simulink model "corner_detection_2019b_modified"  (R2022b)
settings: Solver=FixedStepDiscrete  StartTime=0.0  StopTime=0  RelTol=1e-3  EnableMultiTasking=on
undefined symbols (not defined in the file or in its folder): fspecial, gray, Rec, SDTV
libraries: visionsources x2, visionconversions x1, visionanalysis x1, visiontextngfix x1
settings Model: PacingRate=0.001800  Creator=FxMain  LastModifiedBy=User
settings SolverCC: AlgebraicLoopSolver=TrustRegion
settings DataIOCC: LimitDataPoints=on  SaveFormat=Array  ReturnWorkspaceOutputs=off
settings OptimizationCC: ExpressionDepthLimit=2147483647  LifeSpan=inf
settings DebuggingCC: UnderspecifiedInitializationDetection=Classic  MergeDetectMultiDrivingBlocksExec=none  SolverPrmCheckMsg=warning  FcnCallInpInsideContextMsg=warning  UnconnectedInputMsg=warning  UnconnectedOutputMsg=warning  UnconnectedLineMsg=warning  StateNameClashWarn=warning  SFUnexpectedBacktrackingDiag=warning  SFNoUnconditionalDefaultTransitionDiag=warning  SFExecutionAtInitializationDiag=none  SFMachineParentedDataDiag=warning  ArithmeticOperatorsInVariantConditions=warning
settings HardwareCC: ProdBitPerPointer=32  ProdBitPerSizeT=32  ProdBitPerPtrDiffT=32  ProdLargestAtomicFloat=None  ProdIntDivRoundTo=Undefined  ProdEndianess=Unspecified  ProdWordSize=32  ProdHWDeviceType=32-bit Generic
settings ModelReferenceCC: EnableRefExpFcnMdlSchedulingChecks=on  PropagateSignalLabelsOutOfModel=off
settings SFSimCC: SimUseLocalCustomCode=off  CustomCodeUndefinedFunction=UseInterfaceOnly
settings RTWCC: RTWUseLocalCustomCode=off
settings CodeAppCC: StateflowObjectComments=on
settings GRTTargetCC: TargetLangStandard=C89/C90 (ANSI)  CombineOutputUpdateFcns=off  GRTInterface=on
settings ConfigComp: CovMetricSettings=dw  CovSaveCumulativeToWorkspaceVar=on  CovSaveSingleToWorkspaceVar=on  CovExternalEMLEnable=off

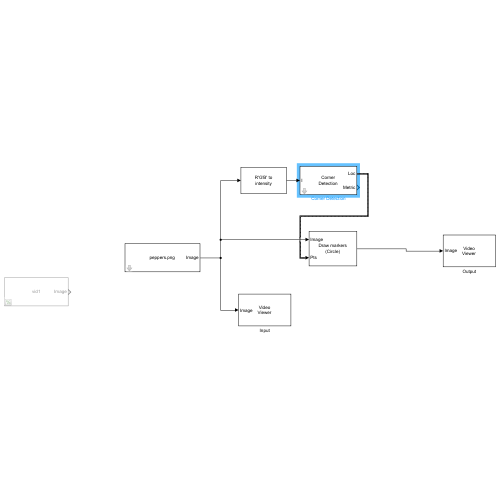
[thumbnail: Simulink's stored preview of the top-level diagram]
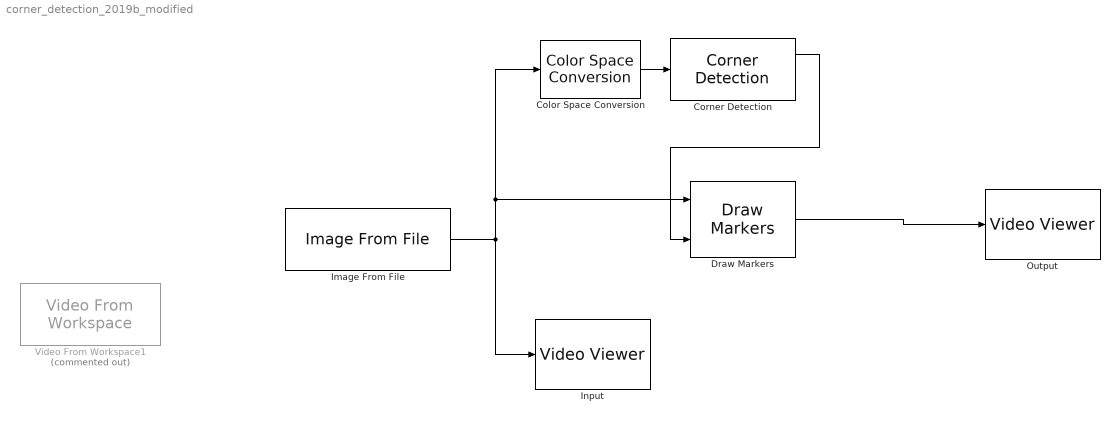
== system corner_detection_2019b_modified ==
  Color Space Conversion : visionconversions/Color Space  Conversion  conversion=Obsolete  conversionActive=R'G'B' to intensity  wp_str=D65  rec=Rec. 601 (SDTV)  sys=1125/60/2:1  imagePorts=One multidimensional signal
  Corner Detection : visionanalysis/Corner Detection  method=Local intensity comparison (Rosen & Drummond)  factor=0.02  filter=fspecial('gaussian', [1 5], 1.5)  thrInten=0.1  thrAngle=157.5  output=Obsolete9b  outputInUse=Corner location and metric matrix  maxNum=300  thrMetric=0.0005  neighborSize=[11 11]  isOutVarDim=on  roundingMode=Floor  overflowMode=off  firstCoeffMode=Specify word length  firstCoeffWordLength=16  firstCoeffFracLength=16  prodOutputMode=Binary point scaling  prodOutputWordLength=32  prodOutputFracLength=0  accumMode=Binary point scaling  accumWordLength=32  accumFracLength=0  memoryMode=Binary point scaling  memoryWordLength=32  memoryFracLength=0
  Draw Markers : visiontextngfix/Draw Markers  shape=Circle  size=20  fill=on  fillClrSource=Specify via dialog  display=White  intensity=200  color=255  opacity=0.6  viewport=Entire image  antialiasing=off  inType=Obsolete  imagePorts=One multidimensional signal  roundingMode=Floor  overflowMode=off  memoryMode=Specify word length  memoryWordLength=16  memoryFracLength=15  prodOutputMode=Binary point scaling  prodOutputWordLength=32  prodOutputFracLength=14
  Image From File : visionsources/Image From File  Tag=vipblks_nd  FileName=peppers.png  Ts=inf  imagePorts=One multidimensional signal  OutPortLabels=R|G|B  ImageDataType=Inherit from input image  sdImageDataType=uint(8)  Signed=on  WordLength=16  FractionLengthMode=User-defined  FractionLength=15
  Input : VideoViewer  colormapValue=gray(256)  FigPos=[141.8 567.6 519.2 385.6]
  Output : VideoViewer  colormapValue=gray(256)  FigPos=[663.4 573.2 520 384.8]
  Video From Workspace1 : visionsources/Video From Workspace  Commented=on  signal=vid1  Ts=1  finalout=Obsolete  finaloutActive=Setting to zero  imagePorts=One multidimensional signal  OutPortLabels=R|G|B
  wires:
  Image From File/1 -> Draw Markers/1, Color Space Conversion/1, Input/1
  Color Space Conversion/1 -> Corner Detection/1
  Corner Detection/1 -> Draw Markers/2
  Draw Markers/1 -> Output/1
